simulink model "nsdynamic_Force1"  (R2021b)
settings: Solver=ode4  StartTime=0.0  StopTime=10.0  RelTol=1e-3
InitFcn:
  | initialization
undefined symbols (not defined in the file or in its folder): dynNS_Force1, trajectory
settings Model: Creator=AzamaoZ  LastModifiedBy=AzamaoZ

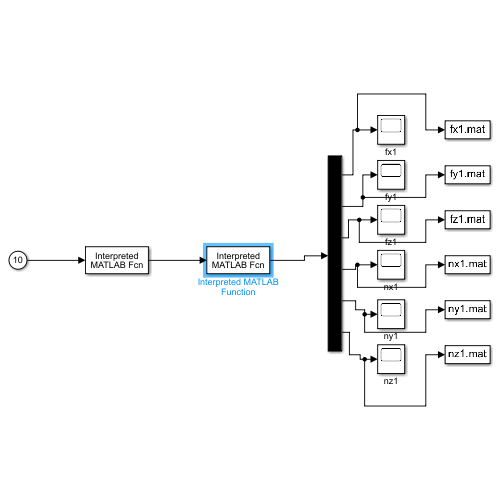
[thumbnail: Simulink's stored preview of the top-level diagram]
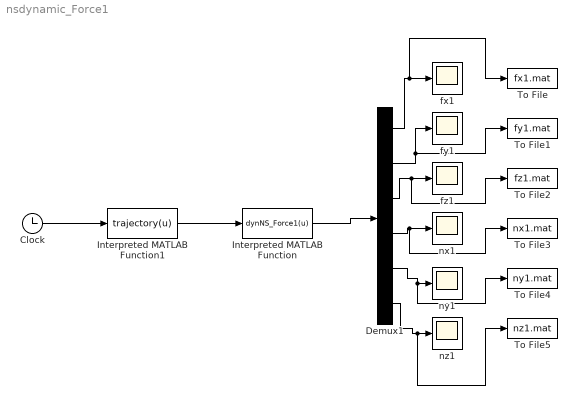
== system nsdynamic_Force1 ==
  Clock : Clock
  Demux1 : Demux  Outputs=6
  Interpreted MATLAB Function : MATLABFcn  MATLABFcn=dynNS_Force1(u)  OutputDimensions=6
  Interpreted MATLAB Function1 : MATLABFcn  MATLABFcn=trajectory(u)
  To File : ToFile  Filename=fx1.mat  MatrixName=fx1  SaveFormat=Timeseries
  To File1 : ToFile  Filename=fy1.mat  MatrixName=fy1  SaveFormat=Timeseries
  To File2 : ToFile  Filename=fz1.mat  MatrixName=fz1  SaveFormat=Timeseries
  To File3 : ToFile  Filename=nx1.mat  MatrixName=nx1  SaveFormat=Timeseries
  To File4 : ToFile  Filename=ny1.mat  MatrixName=ny1  SaveFormat=Timeseries
  To File5 : ToFile  Filename=nz1.mat  MatrixName=nz1  SaveFormat=Timeseries
  fx1 : Scope
  fy1 : Scope
  fz1 : Scope
  nx1 : Scope
  ny1 : Scope
  nz1 : Scope
  wires:
  Interpreted MATLAB Function/1 -> Demux1/1
  Clock/1 -> Interpreted MATLAB Function1/1
  Demux1/2 -> fy1/1, To File1/1
  Demux1/4 -> To File3/1, nx1/1
  Demux1/6 -> To File5/1, nz1/1
  Demux1/5 -> To File4/1, ny1/1
  Demux1/3 -> To File2/1, fz1/1
  Interpreted MATLAB Function1/1 -> Interpreted MATLAB Function/1
  Demux1/1 -> To File/1, fx1/1
